simulink model "HapticPaddleSin"  (Simulink 8.8)
settings: Solver=ode4  StartTime=0.0  StopTime=100.0  FixedStep=0.01  RelTol=1e-3  EnableMultiTasking=on
values from neighbouring files (symbols this model uses):
  B_eq = B_p + B_m * R^2    (= 0.00017775)    [main.m]
  dry_friction = 0.001    [main.m]
  g = 9.81    [main.m]
  J_eq = J_p + (J_rotor+J_m) * R^2    (= 0.0005755)    [main.m]
  l = 0.0199    [main.m]
  m_p = 0.075    [main.m]
  R = r_p1 / r_m    (= 15)    [main.m]
  r_p2 = 0.065    [main.m]
libraries: simulink_extras x3
settings Model: Creator=jemetzge  LastModifiedBy=Hannes
settings OptimizationCC: ExpressionDepthLimit=2147483647
settings DebuggingCC: SolverPrmCheckMsg=warning
settings ConfigComp: CovSFcnEnable=off

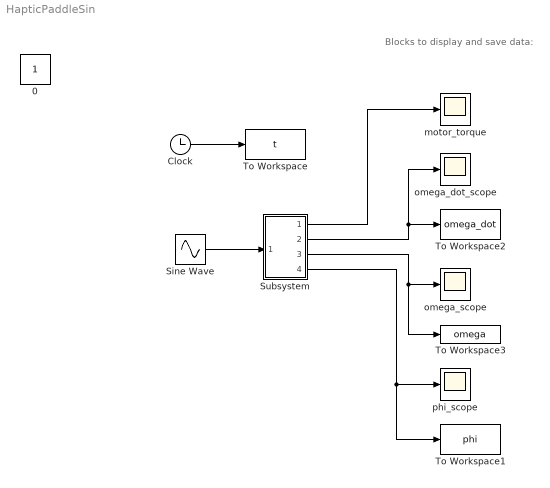
== system HapticPaddleSin ==
  note: Blocks to display and save data:
  Clock : Clock
  Sine Wave : Sin  Amplitude=0.0011  Frequency=2*pi*0.5  SampleTime=0
  Subsystem : Subsystem
  To Workspace : ToWorkspace  VariableName=t  SampleTime=-1
  To Workspace1 : ToWorkspace  VariableName=phi  SampleTime=-1
  To Workspace2 : ToWorkspace  VariableName=omega_dot  SampleTime=-1
  To Workspace3 : ToWorkspace  VariableName=omega  SampleTime=-1
  motor_torque : Scope
  omega_dot_scope : Scope
  omega_scope : Scope
  phi_scope : Scope
  0 : Constant  IOType=siggen
  wires:
  Clock/1 -> To Workspace/1
  Subsystem/4(Out4) -> phi_scope/1, To Workspace1/1
  Subsystem/3(Out3) -> omega_scope/1, To Workspace3/1
  Subsystem/2(Out2) -> omega_dot_scope/1, To Workspace2/1
  Sine Wave/1 -> Subsystem/1(In1)
  Subsystem/1(Out1) -> motor_torque/1

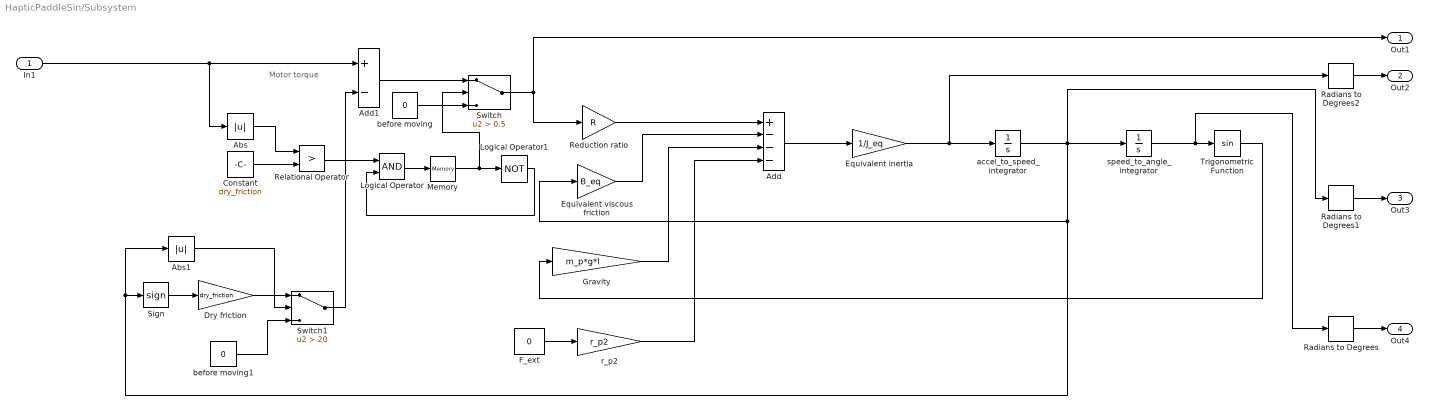
== system HapticPaddleSin/Subsystem ==
  note: Motor torque
  In1 : Inport
  Abs : Abs
  Abs1 : Abs
  Add : Sum  Inputs=+---
  Add1 : Sum  Inputs=+-
  Constant : Constant  Value=dry_friction
  Dry friction : Gain  Gain=dry_friction
  Equivalent inertia : Gain  Gain=1/J_eq
  Equivalent viscous friction : Gain  Gain=B_eq
  F_ext : Constant  Value=0
  Gravity : Gain  Gain=m_p*g*l
  Logical Operator : Logic  AllPortsSameDT=off  OutDataTypeStr=boolean
  Logical Operator1 : Logic  Operator=NOT  Inputs=1  AllPortsSameDT=off  OutDataTypeStr=boolean
  Memory : Memory  InheritSampleTime=on  LinearizeAsDelay=on
  Radians to Degrees : simulink_extras/Transformations/Radians to Degrees
  Radians to Degrees1 : simulink_extras/Transformations/Radians to Degrees
  Radians to Degrees2 : simulink_extras/Transformations/Radians to Degrees
  Reduction ratio : Gain  Gain=R
  Relational Operator : RelationalOperator  Operator=>  OutDataTypeStr=boolean  RndMeth=Simplest
  Sign : Signum
  Switch : Switch  Criteria=u2 > Threshold  Threshold=0.5
  Switch1 : Switch  Criteria=u2 > Threshold  Threshold=20
  Trigonometric Function : Trigonometry
  accel_to_speed_integrator : Integrator
  before moving : Constant  Value=0
  before moving1 : Constant  Value=0
  r_p2 : Gain  Gain=r_p2
  speed_to_angle_integrator : Integrator
  Out1 : Outport
  Out2 : Outport  Port=2
  Out3 : Outport  Port=3
  Out4 : Outport  Port=4
  wires:
  F_ext/1 -> r_p2/1
  Equivalent inertia/1 -> Radians to Degrees2/1, accel_to_speed_integrator/1
  Relational Operator/1 -> Logical Operator/1
  Radians to Degrees1/1 -> Out3/1
  Memory/1 -> Switch/2, Logical Operator1/1
  Add1/1 -> Switch/1
  before moving/1 -> Switch/3
  Logical Operator1/1 -> Logical Operator/2
  accel_to_speed_integrator/1 -> speed_to_angle_integrator/1, Radians to Degrees1/1, Abs1/1, Sign/1, Equivalent viscous friction/1
  Switch1/1 -> Add1/2
  Dry friction/1 -> Switch1/1
  Equivalent viscous friction/1 -> Add/2
  Add/1 -> Equivalent inertia/1
  Radians to Degrees2/1 -> Out2/1
  Sign/1 -> Dry friction/1
  Radians to Degrees/1 -> Out4/1
  Abs1/1 -> Switch1/2
  Trigonometric Function/1 -> Gravity/1
  Switch/1 -> Out1/1, Reduction ratio/1
  r_p2/1 -> Add/4
  Logical Operator/1 -> Memory/1
  Gravity/1 -> Add/3
  Abs/1 -> Relational Operator/1
  before moving1/1 -> Switch1/3
  Reduction ratio/1 -> Add/1
  Constant/1 -> Relational Operator/2
  speed_to_angle_integrator/1 -> Radians to Degrees/1, Trigonometric Function/1
  In1/1 -> Abs/1, Add1/1
